simulink model "3_ZSM"  (R2016a)
settings: Solver=ode1  StartTime=0.0  StopTime=t_sim  FixedStep=0.001  RelTol=1e-3
values from neighbouring files (symbols this model uses):
  A = 1.5    [3_ZSM_Parameters.m]
  C = 1.3    [2_ESM_Parameters.m]    (also in 3_ZSM_Parameters.m)
  c_h_l = 0.5 * c_h    (= 71619.7243914)    [3_ZSM_Parameters.m]
  c_h_r = 0.5 * c_h    (= 71619.7243914)    [3_ZSM_Parameters.m]
  c_v_l = 0.5 * c_v    (= 39054.886799)    [3_ZSM_Parameters.m]
  c_v_r = 0.5 * c_v    (= 39054.886799)    [3_ZSM_Parameters.m]
  c_w = 0.4    [3_ZSM_Parameters.m]
  dynamicload_mode = i-1    [3_ZSM_Parameters.m]
  E = 0.85    [2_ESM_Parameters.m]    (also in 3_ZSM_Parameters.m)
  f_x_init = 0.5*A*c_w*rho*v_init^2    (= 24.980004)    [3_ZSM_Parameters.m]
  fz1 = fz(:,1)    [3_ZSM_Parameters.m]
  g = 9.81    [3_ZSM_Parameters.m]
  h_s = 0.5    [3_ZSM_Parameters.m]
  L = 2.71    [2_ESM_Parameters.m]    (also in 3_ZSM_Parameters.m)
  l_h = m_v * L / m    (= 1.35481930924)    [2_ESM_Parameters.m]    (also in 3_ZSM_Parameters.m)
  l_v = m_h * L / m    (= 1.35518069076)    [2_ESM_Parameters.m]    (also in 3_ZSM_Parameters.m)
  m = m_v + m_h    (= 1499.8)    [2_ESM_Parameters.m]    (also in 3_ZSM_Parameters.m)
  m_hl = m * l_v / L * SP_yl    (= 375)    [3_ZSM_Parameters.m]
  m_hr = m * l_v / L * SP_yr    (= 375)    [3_ZSM_Parameters.m]
  m_vl = m * l_h / L * SP_yl    (= 374.9)    [3_ZSM_Parameters.m]
  m_vr = m * l_h / L * SP_yr    (= 374.9)    [3_ZSM_Parameters.m]
  mu = 0.9    [2_ESM_Parameters.m]    (also in 3_ZSM_Parameters.m)
  rho = 1.2    [3_ZSM_Parameters.m]
  s_h = 1.57    [3_ZSM_Parameters.m]
  s_v = 1.54    [3_ZSM_Parameters.m]
  SP_yl = 0.5    [3_ZSM_Parameters.m]
  SP_yr = 1 - SP_yl    (= 0.5)    [3_ZSM_Parameters.m]
  v = setting(i,3)    [2_ESM_Parameters.m]
  v_init = 8.33    [3_ZSM_Parameters.m]
undefined symbols (not defined in the file or in its folder): Delta, fz
undefined symbols (not defined in the file): Lenkwinkel, Radlenkwinkel, T_z
libraries: simulink x2
(part 1 of 2)
settings Model: Creator=KFZ00  LastModifiedBy=Mario
settings DataIOCC: SaveFormat=Array  SaveOutput=off  TimeSaveName=t_out
settings DebuggingCC: AllowSymbolicDim=off
settings ModelReferenceCC: PropagateSignalLabelsOutOfModel=off
settings GRTTargetCC: GeneratePreprocessorConditionals=Use local settings

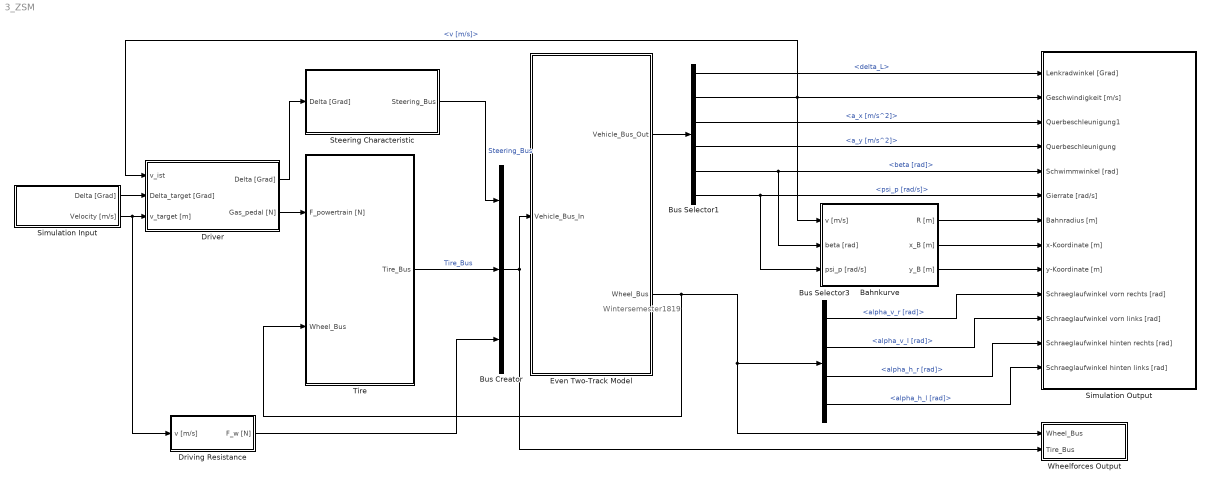
== system 3_ZSM ==
  note: Wintersemester1819
  Bahnkurve : Subsystem
  Bus Creator : BusCreator  Inputs=3
  Bus Selector1 : BusSelector  OutputSignals=delta_L,v [m/s],a_x [m/s^2],a_y [m/s^2],beta [rad],psi_p [rad/s]
  Bus Selector3 : BusSelector  OutputSignals=alpha_v_r [rad],alpha_v_l [rad],alpha_h_r [rad],alpha_h_l [rad]
  Driver : Subsystem
  Driving Resistance : Subsystem
  Even Two-Track Model : Subsystem  mask(Vehicle Model){m_body=m, I_zz_body=T_z, l_front=l_v, l_rear=l_h, tw_front=s_v, tw_rear=s_h, wb=L, h_cog=h_s, g=g}
      mask prompts: m_body "Vehicle Body Mass [kg]"; I_zz_body "Vehicle Body Inertia zz [kgm^2]"; l_front "Distance COG Front Axle [m]"; l_rear "Distance COG Rear Axle [m]"; tw_front "Track Width Front Axle [m]"; tw_rear "Track Width Rear Axle [m]"; wb "Wheelbase [m]"; h_cog "Height COG [m]"; g "Gravity [m/s^2]"
      mask help:
      | Even two-track model without wheel bodies and suspension system.
      |
      | Source for equations:
      | Von Vietinghoff, A.: Nichtlineare Regelung von Kraftfahrzeugen in
      | querdynamisch kritischen Fahrsituationen. Dissertation, Universität
      | Karlsruhe, S. 10 - 33, 2008.
  Simulation Input : Subsystem
  Simulation Output : Subsystem
  Steering Characteristic : Subsystem  mask(Steering Model){Input_values=Lenkwinkel, Steering_angles=Radlenkwinkel}
      mask prompts: Input_values "Steering Input Values [°]"; Steering_angles "Wheel Steer Angles [°]"
      mask help:
      | Steering model uses a look-up table to determine the current wheel
      | steer angle.
      | The steering angle of the rear wheel is set to zero!
      |
      | In order to configure the look-up table define the input values (steering
      | wheel angle in °) and the corresponding wheel steer angles (in °).
  Tire : Subsystem
  Wheelforces Output : Subsystem
  wires:
  Driver/1(Delta [Grad]) -> Steering Characteristic/1(Delta [Grad])
  Bus Creator/1 -> Even Two-Track Model/1(Vehicle_Bus_In), Wheelforces Output/2(Tire_Bus)
  Steering Characteristic/1(Steering_Bus) -> Bus Creator/1  "Steering_Bus"
  Tire/1(Tire_Bus) -> Bus Creator/2  "Tire_Bus"
  Even Two-Track Model/2(Wheel_Bus) -> Tire/2(Wheel_Bus), Bus Selector3/1, Wheelforces Output/1(Wheel_Bus)
  Even Two-Track Model/1(Vehicle_Bus_Out) -> Bus Selector1/1
  Bus Selector1/2 -> Bahnkurve/1(v [m/s]), Simulation Output/2(Geschwindigkeit [m/s]), Driver/1(v_ist)  "<v [m/s]>"
  Bus Selector1/4 -> Simulation Output/4(Querbeschleunigung)  "<a_y [m/s^2]>"
  Bus Selector1/5 -> Bahnkurve/2(beta [rad]), Simulation Output/5(Schwimmwinkel [rad])  "<beta [rad]>"
  Bus Selector1/6 -> Bahnkurve/3(psi_p [rad/s]), Simulation Output/6(Gierrate [rad/s])  "<psi_p [rad/s]>"
  Bus Selector3/1 -> Simulation Output/10(Schraeglaufwinkel vorn rechts [rad])  "<alpha_v_r [rad]>"
  Bus Selector3/2 -> Simulation Output/11(Schraeglaufwinkel vorn links [rad])  "<alpha_v_l [rad]>"
  Bus Selector3/3 -> Simulation Output/12(Schraeglaufwinkel hinten rechts [rad])  "<alpha_h_r [rad]>"
  Bus Selector3/4 -> Simulation Output/13(Schraeglaufwinkel hinten links [rad])  "<alpha_h_l [rad]>"
  Driving Resistance/1(F_w [N]) -> Bus Creator/3
  Bahnkurve/2(x_B [m]) -> Simulation Output/8(x-Koordinate [m])
  Bahnkurve/3(y_B [m]) -> Simulation Output/9(y-Koordinate [m])
  Bahnkurve/1(R [m]) -> Simulation Output/7(Bahnradius [m])
  Driver/2(Gas_pedal [N]) -> Tire/1(F_powertrain [N])
  Simulation Input/1(Delta [Grad]) -> Driver/2(Delta_target [Grad])
  Simulation Input/2(Velocity [m/s]) -> Driving Resistance/1(v [m/s]), Driver/3(v_target [m])
  Bus Selector1/1 -> Simulation Output/1(Lenkradwinkel [Grad])  "<delta_L>"
  Bus Selector1/3 -> Simulation Output/3(Querbeschleunigung1)  "<a_x [m/s^2]>"

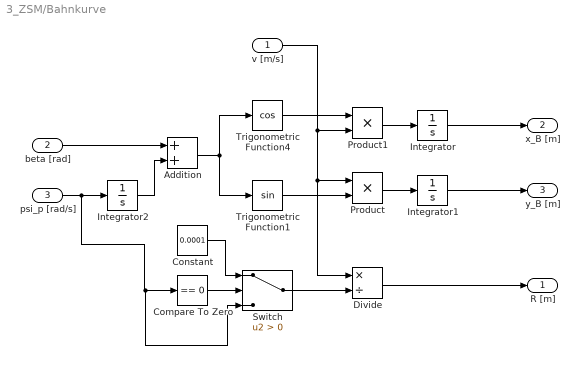
== system 3_ZSM/Bahnkurve ==
  v [m/s] : Inport
  beta [rad] : Inport  Port=2
  psi_p [rad/s] : Inport  Port=3
  Addition : Sum
  Compare To Zero : simulink/Logic and Bit Operations/Compare To Zero  relop===  OutDataTypeStr=boolean
  Constant : Constant  Value=0.0001
  Divide : Product  Inputs=*/
  Integrator : Integrator
  Integrator1 : Integrator
  Integrator2 : Integrator
  Product : Product
  Product1 : Product
  Switch : Switch  Criteria=u2 > Threshold
  Trigonometric Function1 : Trigonometry
  Trigonometric Function4 : Trigonometry  Operator=cos
  R [m] : Outport
  x_B [m] : Outport  Port=2
  y_B [m] : Outport  Port=3
  wires:
  Trigonometric Function4/1 -> Product1/1
  Trigonometric Function1/1 -> Product/2
  Product/1 -> Integrator1/1
  Addition/1 -> Trigonometric Function1/1, Trigonometric Function4/1
  psi_p [rad/s]/1 -> Integrator2/1, Switch/3, Compare To Zero/1
  Integrator2/1 -> Addition/2
  Product1/1 -> Integrator/1
  v [m/s]/1 -> Divide/1, Product/1, Product1/2
  Integrator/1 -> x_B [m]/1
  Integrator1/1 -> y_B [m]/1
  beta [rad]/1 -> Addition/1
  Switch/1 -> Divide/2
  Compare To Zero/1 -> Switch/2
  Divide/1 -> R [m]/1
  Constant/1 -> Switch/1

== system 3_ZSM/Driver ==
  v_ist : Inport
  Delta_target [Grad] : Inport  Port=2
  v_target [m] : Inport  Port=3
  Constant : Constant  Value=f_x_init
  P_Fx : simulink/Continuous/PID Controller (2DOF)  Controller=PI  TimeDomain=Continuous-time  SampleTime=-1  IntegratorMethod=Forward Euler  FilterMethod=Forward Euler  Form=Parallel  UseFilter=on  ControllerParametersSource=internal  P=100000  I=0  D=0  N=100  b=1  c=1  InitialConditionSource=external  InitialConditionForIntegrator=0  InitialConditionForFilter=0  ExternalReset=none  LimitOutput=off  UpperSaturationLimit=9000  LowerSaturationLimit=0  LinearizeAsGain=on  AntiWindupMode=none  Kb=1  TrackingMode=off  Kt=1  PParamMin=[]  PParamMax=[]  IParamMin=[]  IParamMax=[]  DParamMin=[]  DParamMax=[]  NParamMin=[]  NParamMax=[]  bParamMin=[]  bParamMax=[]  cParamMin=[]  cParamMax=[]  KbParamMin=[]  KbParamMax=[]  KtParamMin=[]  KtParamMax=[]  POutMin=[]  POutMax=[]  IOutMin=[]  IOutMax=[]  DOutMin=[]  DOutMax=[]  NOutMin=[]  NOutMax=[]  bOutMin=[]  bOutMax=[]  cOutMin=[]  cOutMax=[]  KbOutMin=[]  KbOutMax=[]  KtOutMin=[]  KtOutMax=[]  IntegratorOutMin=[]  IntegratorOutMax=[]  FilterOutMin=[]  FilterOutMax=[]  SumOutMin=[]  SumOutMax=[]  Sum1OutMin=[]  Sum1OutMax=[]  Sum2OutMin=[]  Sum2OutMax=[]  Sum3OutMin=[]  Sum3OutMax=[]  SumI1OutMin=[]  SumI1OutMax=[]  SumI2OutMin=[]  SumI2OutMax=[]  SumI3OutMin=[]  SumI3OutMax=[]  SumDOutMin=[]  SumDOutMax=[]  SaturationOutMin=[]  SaturationOutMax=[]  IntegratorContinuousStateAttributes=''  IntegratorStateMustResolveToSignalObject=off  IntegratorRTWStateStorageClass=Auto  FilterContinuousStateAttributes=''  FilterStateMustResolveToSignalObject=off  FilterRTWStateStorageClass=Auto  DifferentiatorICPrevScaledInput=0  DifferentiatorOutMin=[]  DifferentiatorOutMax=[]
  Scope : Scope  NumInputPorts=2
  Delta [Grad] : Outport
  Gas_pedal [N] : Outport  Port=2
  wires:
  v_target [m]/1 -> Scope/1, P_Fx/1
  Constant/1 -> P_Fx/3
  P_Fx/1 -> Gas_pedal [N]/1
  v_ist/1 -> Scope/2, P_Fx/2
  Delta_target [Grad]/1 -> Delta [Grad]/1

== system 3_ZSM/Driving Resistance ==
  v [m/s] : Inport
  Constant : Constant  Value=c_w
  Constant1 : Constant  Value=A
  Constant2 : Constant  Value=rho
  Constant3 : Constant  Value=0.5
  Math Function : Math  Operator=square  SaturateOnIntegerOverflow=on
  Product : Product  Inputs=5
  F_w [N] : Outport
  wires:
  Constant3/1 -> Product/5
  Product/1 -> F_w [N]/1  "Driving_resistance [N]"
  Constant2/1 -> Product/4
  Constant/1 -> Product/1
  v [m/s]/1 -> Math Function/1
  Math Function/1 -> Product/3
  Constant1/1 -> Product/2

== system 3_ZSM/Even Two-Track Model ==
  Vehicle_Bus_In : Inport
  Bus Creator1 : BusCreator  Inputs=8
  Bus Creator2 : BusCreator  Inputs=6
  Bus Selector : BusSelector  OutputSignals=Steering_Bus.delta_L
  Calculate Wheel Load : Subsystem
  Calculate forces on vehicle body : Subsystem
  Calculate side slip angle : Subsystem
  Calculate sum of forces (x and y) : Subsystem
  Calculate velocity : Subsystem
  Calculate yaw rate : Subsystem
  Determine vehicle body movement in vehicle COS : Subsystem
  Determine wheel movement : Subsystem
  Scope : Scope
  Vehicle_Bus_Out : Outport
  Wheel_Bus : Outport  Port=2
  wires:
  Calculate velocity/1(v [m/s]) -> Determine vehicle body movement in vehicle COS/1(v [m/s]), Calculate side slip angle/1(v [m/s]), Bus Creator2/3, Determine wheel movement/1(vehicle_velocity [m/s])  "v [m/s]"
  Determine vehicle body movement in vehicle COS/2(a_y [m/s^2]) -> Calculate Wheel Load/2(a_y [m/s²]), Bus Creator2/2  "a_y [m/s^2]"
  Calculate side slip angle/2(beta_p [rad/s]) -> Scope/1, Determine vehicle body movement in vehicle COS/4(beta_p [rad/s])
  Calculate velocity/2(v_p [m/s^2]) -> Determine vehicle body movement in vehicle COS/2(v_p [m/s^2])
  Calculate sum of forces (x and y)/2(Sum_F_y [N]) -> Calculate velocity/2(Sum_F_y [N]), Calculate side slip angle/3(Sum_F_y [N])
  Calculate sum of forces (x and y)/1(Sum_F_x [N]) -> Calculate side slip angle/2(Sum_F_x [N]), Calculate velocity/1(Sum_F_x [N])
  Calculate side slip angle/1(Side_slip_angle [rad]) -> Determine vehicle body movement in vehicle COS/3(beta [rad]), Calculate side slip angle/4(beta [rad]), Calculate velocity/3(beta [rad]), Bus Creator2/4, Determine wheel movement/2(beta [rad])  "beta [rad]"
  Calculate forces on vehicle body/1(Forces_vehicle_COS [N]) -> Calculate sum of forces (x and y)/1(Forces_vehicle_body [N]), Calculate yaw rate/1(Forces_vehicle_body [N])
  Calculate yaw rate/1(psi_p [rad/s]) -> Determine vehicle body movement in vehicle COS/5(psi_p [rad/s]), Calculate side slip angle/5(psi_p [rad]), Bus Creator2/5, Determine wheel movement/3(psi_p [rad/s])  "psi_p [rad/s]"
  Vehicle_Bus_In/1 -> Calculate forces on vehicle body/1(Vehicle Bus), Determine wheel movement/4(Vehicle Bus In), Bus Selector/1
  Bus Creator1/1 -> Wheel_Bus/1
  Bus Creator2/1 -> Vehicle_Bus_Out/1
  Determine vehicle body movement in vehicle COS/1(a_x [m/s^2]) -> Bus Creator2/1, Calculate Wheel Load/1(a_x [m/s²])  "a_x [m/s^2]"
  Calculate Wheel Load/1(F_z_v_l [N]) -> Bus Creator1/1  "F_z_v_l [N]"
  Calculate Wheel Load/2(F_z_v_r [N]) -> Bus Creator1/2  "F_z_v_r [N]"
  Calculate Wheel Load/3(F_z_h_l [N]) -> Bus Creator1/3  "F_z_h_l [N]"
  Calculate Wheel Load/4(F_z_h_r [N]) -> Bus Creator1/4  "F_z_h_r [N]"
  Determine wheel movement/4(alpha_rear_left [rad]) -> Bus Creator1/8  "alpha_h_l [rad]"
  Determine wheel movement/3(alpha_rear_right [rad]) -> Bus Creator1/7  "alpha_h_r [rad]"
  Determine wheel movement/2(alpha_front_left [rad]) -> Bus Creator1/6  "alpha_v_l [rad]"
  Determine wheel movement/1(alpha_front_right [rad]) -> Bus Creator1/5  "alpha_v_r [rad]"
  Bus Selector/1 -> Bus Creator2/6  "<delta_L>"

== system 3_ZSM/Simulation Input ==
  1-D Lookup Table : Lookup_n-D  NumberOfTableDimensions=1  BreakpointsForDimension1=Delta.time  Table=Delta.signals.values  InternalRulePriority=Speed  RndMeth=Simplest  InputSameDT=on
  1-D Lookup Table1 : Lookup_n-D  NumberOfTableDimensions=1  BreakpointsForDimension1=v.time  Table=v.signals.values  InternalRulePriority=Speed  RndMeth=Simplest  InputSameDT=on
  Clock : Clock
  Gain : Gain  Gain=1/3.6
  Delta [Grad] : Outport
  Velocity [m/s] : Outport  Port=2
  wires:
  Clock/1 -> 1-D Lookup Table/1, 1-D Lookup Table1/1
  1-D Lookup Table/1 -> Delta [Grad]/1
  1-D Lookup Table1/1 -> Gain/1
  Gain/1 -> Velocity [m/s]/1

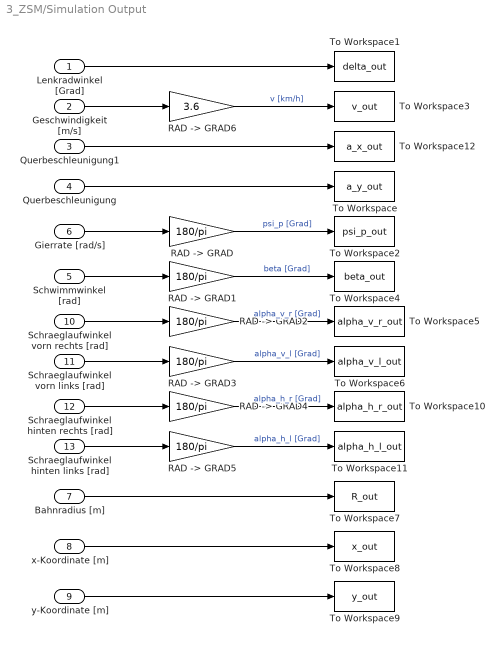
== system 3_ZSM/Simulation Output ==
  Lenkradwinkel [Grad] : Inport
  Geschwindigkeit [m/s] : Inport  Port=2
  Querbeschleunigung1 : Inport  Port=3
  Querbeschleunigung : Inport  Port=4
  Schwimmwinkel [rad] : Inport  Port=5
  Gierrate [rad/s] : Inport  Port=6
  Bahnradius [m] : Inport  Port=7
  x-Koordinate [m] : Inport  Port=8
  y-Koordinate [m] : Inport  Port=9
  Schraeglaufwinkel vorn rechts [rad] : Inport  Port=10
  Schraeglaufwinkel vorn links [rad] : Inport  Port=11
  Schraeglaufwinkel hinten rechts [rad] : Inport  Port=12
  Schraeglaufwinkel hinten links [rad] : Inport  Port=13
  RAD -> GRAD{,1..5} (6 alike) : Gain  Gain=180/pi
  "RAD -> GRAD6" : Gain  Gain=3.6
  To Workspace : ToWorkspace  VariableName=a_y_out  SampleTime=-1
      settings: Save2DSignal=2-D array (concatenate along first dimension)
  To Workspace1 : ToWorkspace  VariableName=delta_out  SampleTime=-1
      settings: Save2DSignal=2-D array (concatenate along first dimension)
  To Workspace10 : ToWorkspace  VariableName=alpha_h_r_out  SampleTime=-1
      settings: Save2DSignal=2-D array (concatenate along first dimension)
  To Workspace11 : ToWorkspace  VariableName=alpha_h_l_out  SampleTime=-1
      settings: Save2DSignal=2-D array (concatenate along first dimension)
  To Workspace12 : ToWorkspace  VariableName=a_x_out  SampleTime=-1
      settings: Save2DSignal=2-D array (concatenate along first dimension)
  To Workspace2 : ToWorkspace  VariableName=psi_p_out  SampleTime=-1
      settings: Save2DSignal=2-D array (concatenate along first dimension)
  To Workspace3 : ToWorkspace  VariableName=v_out  SampleTime=-1
      settings: Save2DSignal=2-D array (concatenate along first dimension)
  To Workspace4 : ToWorkspace  VariableName=beta_out  SampleTime=-1
      settings: Save2DSignal=2-D array (concatenate along first dimension)
  To Workspace5 : ToWorkspace  VariableName=alpha_v_r_out  SampleTime=-1
      settings: Save2DSignal=2-D array (concatenate along first dimension)
  To Workspace6 : ToWorkspace  VariableName=alpha_v_l_out  SampleTime=-1
      settings: Save2DSignal=2-D array (concatenate along first dimension)
  To Workspace7 : ToWorkspace  VariableName=R_out  SampleTime=-1
      settings: Save2DSignal=2-D array (concatenate along first dimension)
  To Workspace8 : ToWorkspace  VariableName=x_out  SampleTime=-1
      settings: Save2DSignal=2-D array (concatenate along first dimension)
  To Workspace9 : ToWorkspace  VariableName=y_out  SampleTime=-1
      settings: Save2DSignal=2-D array (concatenate along first dimension)
  wires:
  Gierrate [rad/s]/1 -> "RAD -> GRAD"/1
  "RAD -> GRAD"/1 -> To Workspace2/1  "psi_p [Grad]"
  Lenkradwinkel [Grad]/1 -> To Workspace1/1
  Geschwindigkeit [m/s]/1 -> "RAD -> GRAD6"/1
  Schwimmwinkel [rad]/1 -> "RAD -> GRAD1"/1
  "RAD -> GRAD1"/1 -> To Workspace4/1  "beta [Grad]"
  Schraeglaufwinkel vorn rechts [rad]/1 -> "RAD -> GRAD2"/1
  "RAD -> GRAD2"/1 -> To Workspace5/1  "alpha_v_r [Grad]"
  Schraeglaufwinkel vorn links [rad]/1 -> "RAD -> GRAD3"/1
  "RAD -> GRAD3"/1 -> To Workspace6/1  "alpha_v_l [Grad]"
  Bahnradius [m]/1 -> To Workspace7/1
  x-Koordinate [m]/1 -> To Workspace8/1
  y-Koordinate [m]/1 -> To Workspace9/1
  Schraeglaufwinkel hinten rechts [rad]/1 -> "RAD -> GRAD4"/1
  "RAD -> GRAD4"/1 -> To Workspace10/1  "alpha_h_r [Grad]"
  Schraeglaufwinkel hinten links [rad]/1 -> "RAD -> GRAD5"/1
  "RAD -> GRAD5"/1 -> To Workspace11/1  "alpha_h_l [Grad]"
  "RAD -> GRAD6"/1 -> To Workspace3/1  "v [km/h]"
  Querbeschleunigung/1 -> To Workspace/1
  Querbeschleunigung1/1 -> To Workspace12/1

== system 3_ZSM/Steering Characteristic ==
  Delta [Grad] : Inport  OutDataTypeStr=double
  1-D Lookup Table : Lookup_n-D  NumberOfTableDimensions=1  BreakpointsForDimension1=Input_values  Table=Steering_angles  InternalRulePriority=Speed  RndMeth=Simplest  InputSameDT=on
  Bus Creator : BusCreator  Inputs=5
  "Grad -> RAD1" : Gain  Gain=pi/180
  "Grad -> RAD2" : Gain  Gain=pi/180
  Rear wheel steering left : Constant  Value=0
  Rear wheel steering right : Constant  Value=0
  Steering_Bus : Outport  OutDataTypeStr=double
  wires:
  Bus Creator/1 -> Steering_Bus/1
  1-D Lookup Table/1 -> "Grad -> RAD1"/1, "Grad -> RAD2"/1
  "Grad -> RAD1"/1 -> Bus Creator/1  "Delta_v_l"
  "Grad -> RAD2"/1 -> Bus Creator/2  "Delta_v_r"
  Rear wheel steering left/1 -> Bus Creator/3  "Delta_h_l"
  Rear wheel steering right/1 -> Bus Creator/4  "Delta_h_r"
  Delta [Grad]/1 -> Bus Creator/5, 1-D Lookup Table/1  "delta_L"

== system 3_ZSM/Tire ==
  F_powertrain [N] : Inport
  Wheel_Bus : Inport  Port=2
  Bus Creator : BusCreator  Inputs=4
  Constant : Constant  Value=mu
  Constant1 : Constant  Value=0
  Gain : Gain  Gain=1/2
  Tire front left : Subsystem
  Tire front right : Subsystem
  Tire rear left : Subsystem
  Tire rear right : Subsystem
  Tire_Bus : Outport
  wires:
  F_powertrain [N]/1 -> Gain/1
  Bus Creator/1 -> Tire_Bus/1
  Wheel_Bus/1 -> Tire rear right/2(Wheel_Bus), Tire rear left/2(Wheel_Bus), Tire front right/2(Wheel_Bus), Tire front left/2(Wheel_Bus)
  Tire rear right/1(Tire_front_left) -> Bus Creator/4  "Tire_rear_right"
  Tire rear left/1(Tire_rear_left) -> Bus Creator/3  "Tire_rear_left"
  Tire front right/1(Tire_front_right) -> Bus Creator/2  "Tire_front_right"
  Tire front left/1(Tire_front_left) -> Bus Creator/1  "Tire_front_left"
  Constant/1 -> Tire front right/3(nu_v_r [-]), Tire rear left/3(nu_h_l [-]), Tire rear right/3(nu_h_r [-]), Tire front left/3(nu_v_l [-])
  Constant1/1 -> Tire rear left/1(F_powertrain [N]), Tire rear right/1(F_powertrain [N])
  Gain/1 -> Tire front right/1(F_powertrain [N]), Tire front left/1(F_powertrain [N])

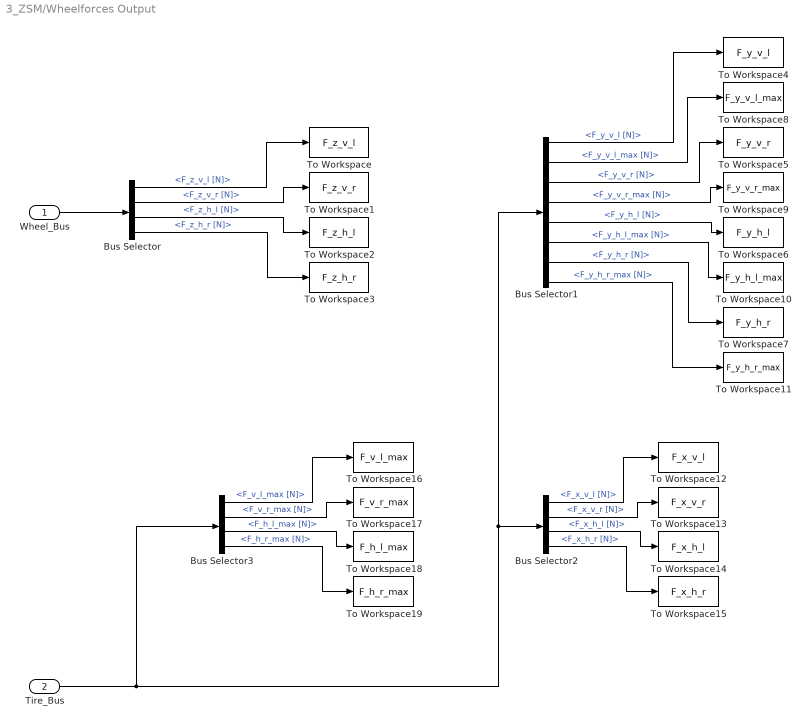
== system 3_ZSM/Wheelforces Output ==
  Wheel_Bus : Inport
  Tire_Bus : Inport  Port=2
  Bus Selector : BusSelector  OutputSignals=F_z_v_l [N],F_z_v_r [N],F_z_h_l [N],F_z_h_r [N]
  Bus Selector1 : BusSelector  OutputSignals=Tire_Bus.Tire_front_left.F_y_v_l [N],Tire_Bus.Tire_front_left.F_y_v_l_max [N],Tire_Bus.Tire_front_right.F_y_v_r [N],Tire_Bus.Tire_front_right.F_y_v_r_max [N],Tire_Bus.Tire_rear_left.F_y_h_l [N],Tire_Bus.Tire_rear_left.F_y_h_l_max [N],Tire_Bus.Tire_rear_right.F_y_h_r [N],Tire_Bus.Tire_rear_right.F_y_h_r_max [N]
  Bus Selector2 : BusSelector  OutputSignals=Tire_Bus.Tire_front_left.F_x_v_l [N],Tire_Bus.Tire_front_right.F_x_v_r [N],Tire_Bus.Tire_rear_left.F_x_h_l [N],Tire_Bus.Tire_rear_right.F_x_h_r [N]
  Bus Selector3 : BusSelector  OutputSignals=Tire_Bus.Tire_front_left.F_v_l_max [N],Tire_Bus.Tire_front_right.F_v_r_max [N],Tire_Bus.Tire_rear_left.F_h_l_max [N],Tire_Bus.Tire_rear_right.F_h_r_max [N]
  To Workspace : ToWorkspace  VariableName=F_z_v_l  SampleTime=-1
      settings: Save2DSignal=2-D array (concatenate along first dimension)
  To Workspace1 : ToWorkspace  VariableName=F_z_v_r  SampleTime=-1
      settings: Save2DSignal=2-D array (concatenate along first dimension)
  To Workspace10 : ToWorkspace  VariableName=F_y_h_l_max  SampleTime=-1
      settings: Save2DSignal=2-D array (concatenate along first dimension)
  To Workspace11 : ToWorkspace  VariableName=F_y_h_r_max  SampleTime=-1
      settings: Save2DSignal=2-D array (concatenate along first dimension)
  To Workspace12 : ToWorkspace  VariableName=F_x_v_l  SampleTime=-1
      settings: Save2DSignal=2-D array (concatenate along first dimension)
  To Workspace13 : ToWorkspace  VariableName=F_x_v_r  SampleTime=-1
      settings: Save2DSignal=2-D array (concatenate along first dimension)
  To Workspace14 : ToWorkspace  VariableName=F_x_h_l  SampleTime=-1
      settings: Save2DSignal=2-D array (concatenate along first dimension)
  To Workspace15 : ToWorkspace  VariableName=F_x_h_r  SampleTime=-1
      settings: Save2DSignal=2-D array (concatenate along first dimension)
  To Workspace16 : ToWorkspace  VariableName=F_v_l_max  SampleTime=-1
      settings: Save2DSignal=2-D array (concatenate along first dimension)
  To Workspace17 : ToWorkspace  VariableName=F_v_r_max  SampleTime=-1
      settings: Save2DSignal=2-D array (concatenate along first dimension)
  To Workspace18 : ToWorkspace  VariableName=F_h_l_max  SampleTime=-1
      settings: Save2DSignal=2-D array (concatenate along first dimension)
  To Workspace19 : ToWorkspace  VariableName=F_h_r_max  SampleTime=-1
      settings: Save2DSignal=2-D array (concatenate along first dimension)
  To Workspace2 : ToWorkspace  VariableName=F_z_h_l  SampleTime=-1
      settings: Save2DSignal=2-D array (concatenate along first dimension)
  To Workspace3 : ToWorkspace  VariableName=F_z_h_r  SampleTime=-1
      settings: Save2DSignal=2-D array (concatenate along first dimension)
  To Workspace4 : ToWorkspace  VariableName=F_y_v_l  SampleTime=-1
      settings: Save2DSignal=2-D array (concatenate along first dimension)
  To Workspace5 : ToWorkspace  VariableName=F_y_v_r  SampleTime=-1
      settings: Save2DSignal=2-D array (concatenate along first dimension)
  To Workspace6 : ToWorkspace  VariableName=F_y_h_l  SampleTime=-1
      settings: Save2DSignal=2-D array (concatenate along first dimension)
  To Workspace7 : ToWorkspace  VariableName=F_y_h_r  SampleTime=-1
      settings: Save2DSignal=2-D array (concatenate along first dimension)
  To Workspace8 : ToWorkspace  VariableName=F_y_v_l_max  SampleTime=-1
      settings: Save2DSignal=2-D array (concatenate along first dimension)
  To Workspace9 : ToWorkspace  VariableName=F_y_v_r_max  SampleTime=-1
      settings: Save2DSignal=2-D array (concatenate along first dimension)
  wires:
  Wheel_Bus/1 -> Bus Selector/1
  Bus Selector/1 -> To Workspace/1  "<F_z_v_l [N]>"
  Bus Selector/2 -> To Workspace1/1  "<F_z_v_r [N]>"
  Bus Selector/3 -> To Workspace2/1  "<F_z_h_l [N]>"
  Bus Selector/4 -> To Workspace3/1  "<F_z_h_r [N]>"
  Bus Selector1/1 -> To Workspace4/1  "<F_y_v_l [N]>"
  Bus Selector1/7 -> To Workspace7/1  "<F_y_h_r [N]>"
  Bus Selector1/3 -> To Workspace5/1  "<F_y_v_r [N]>"
  Bus Selector1/4 -> To Workspace9/1  "<F_y_v_r_max [N]>"
  Bus Selector1/8 -> To Workspace11/1  "<F_y_h_r_max [N]>"
  Bus Selector1/2 -> To Workspace8/1  "<F_y_v_l_max [N]>"
  Bus Selector1/5 -> To Workspace6/1  "<F_y_h_l [N]>"
  Bus Selector1/6 -> To Workspace10/1  "<F_y_h_l_max [N]>"
  Tire_Bus/1 -> Bus Selector3/1, Bus Selector2/1, Bus Selector1/1
  Bus Selector2/1 -> To Workspace12/1  "<F_x_v_l [N]>"
  Bus Selector2/2 -> To Workspace13/1  "<F_x_v_r [N]>"
  Bus Selector2/3 -> To Workspace14/1  "<F_x_h_l [N]>"
  Bus Selector2/4 -> To Workspace15/1  "<F_x_h_r [N]>"
  Bus Selector3/1 -> To Workspace16/1  "<F_v_l_max [N]>"
  Bus Selector3/2 -> To Workspace17/1  "<F_v_r_max [N]>"
  Bus Selector3/3 -> To Workspace18/1  "<F_h_l_max [N]>"
  Bus Selector3/4 -> To Workspace19/1  "<F_h_r_max [N]>"

== system 3_ZSM/Even Two-Track Model/Calculate Wheel Load ==
  a_x [m/s²] : Inport
  a_y [m/s²] : Inport  Port=2
  Dynamic Wheel Load : Subsystem
  Load_Mode : Constant  Value=dynamicload_mode
  Scope : Scope
  Static Wheel Load : Subsystem
  Switch{,1..3} (4 alike) : Switch  Criteria=u2 > Threshold
  F_z_v_l [N] : Outport
  F_z_v_r [N] : Outport  Port=2
  F_z_h_l [N] : Outport  Port=3
  F_z_h_r [N] : Outport  Port=4
  wires:
  a_x [m/s²]/1 -> Dynamic Wheel Load/1(a_x [m/s²])
  a_y [m/s²]/1 -> Dynamic Wheel Load/2(a_y [m/s²])
  Switch/1 -> Scope/1, F_z_v_l [N]/1
  Switch1/1 -> F_z_v_r [N]/1
  Switch2/1 -> F_z_h_l [N]/1
  Switch3/1 -> F_z_h_r [N]/1
  Dynamic Wheel Load/1(F_z_v_l [N]) -> Switch/1
  Dynamic Wheel Load/2(F_z_v_r [N]) -> Switch1/1
  Dynamic Wheel Load/3(F_z_h_l [N]) -> Switch2/1
  Dynamic Wheel Load/4(F_z_h_r [N]) -> Switch3/1
  Static Wheel Load/1(F_z_v_l [N]) -> Switch/3
  Static Wheel Load/2(F_z_v_r [N]) -> Switch1/3
  Static Wheel Load/3(F_z_h_l [N]) -> Switch2/3
  Static Wheel Load/4(F_z_h_r [N]) -> Switch3/3
  Load_Mode/1 -> Switch1/2, Switch3/2, Switch2/2, Switch/2

== system 3_ZSM/Even Two-Track Model/Calculate forces on vehicle body ==
  Vehicle Bus : Inport
  Bus Creator1 : BusCreator  Inputs=9
  Bus Selector : BusSelector  OutputSignals=Driving_resistance [N],Tire_Bus.Tire_front_right,Steering_Bus.Delta_v_r,Tire_Bus.Tire_front_left,Steering_Bus.Delta_v_l,Tire_Bus.Tire_rear_right,Steering_Bus.Delta_h_r,Tire_Bus.Tire_rear_left,Steering_Bus.Delta_h_l
  Bus Selector1 : BusSelector  OutputSignals=F_x_v_r [N],F_y_v_r [N]
  Bus Selector2 : BusSelector  OutputSignals=F_x_v_l [N],F_y_v_l [N]
  Bus Selector3 : BusSelector  OutputSignals=F_x_h_r [N],F_y_h_r [N]
  Bus Selector4 : BusSelector  OutputSignals=F_x_h_l [N],F_y_h_l [N]
  Transform Wheel-COS to Vehicle-COS (front left) : Subsystem
  Transform Wheel-COS to Vehicle-COS (front right) : Subsystem
  Transform Wheel-COS to Vehicle-COS (rear left) : Subsystem
  Transform Wheel-COS to Vehicle-COS (rear right) : Subsystem
  Forces_vehicle_COS [N] : Outport
  wires:
  Vehicle Bus/1 -> Bus Selector/1
  Bus Creator1/1 -> Forces_vehicle_COS [N]/1
  Bus Selector1/1 -> Transform Wheel-COS to Vehicle-COS (front right)/1(F_x_wheel_COS [N])  "<F_x_v_r [N]>"
  Transform Wheel-COS to Vehicle-COS (front left)/1(F_x_vehicle_COS [N]) -> Bus Creator1/4  "F_x_front_left [N]"
  Bus Selector4/2 -> Transform Wheel-COS to Vehicle-COS (rear left)/2(F_y_wheel_COS [N])  "<F_y_h_l [N]>"
  Transform Wheel-COS to Vehicle-COS (rear left)/2(F_y_vehicle_COS [N]) -> Bus Creator1/9  "F_y_rear_left [N]"
  Bus Selector/9 -> Transform Wheel-COS to Vehicle-COS (rear left)/3(Wheel_steering_angle [rad])  "<Delta_h_l>"
  Bus Selector/2 -> Bus Selector1/1  "<Tire_front_right>"
  Bus Selector4/1 -> Transform Wheel-COS to Vehicle-COS (rear left)/1(F_x_wheel_COS [N])  "<F_x_h_l [N]>"
  Bus Selector3/1 -> Transform Wheel-COS to Vehicle-COS (rear right)/1(F_x_wheel_COS [N])  "<F_x_h_r [N]>"
  Transform Wheel-COS to Vehicle-COS (rear right)/2(F_y_vehicle_COS [N]) -> Bus Creator1/7  "F_y_rear_right [N]"
  Bus Selector/7 -> Transform Wheel-COS to Vehicle-COS (rear right)/3(Wheel_steering_angle [rad])  "<Delta_h_r>"
  Bus Selector/4 -> Bus Selector2/1  "<Tire_front_left>"
  Transform Wheel-COS to Vehicle-COS (front left)/2(F_y_vehicle_COS [N]) -> Bus Creator1/5  "F_y_front_left [N]"
  Bus Selector3/2 -> Transform Wheel-COS to Vehicle-COS (rear right)/2(F_y_wheel_COS [N])  "<F_y_h_r [N]>"
  Bus Selector/5 -> Transform Wheel-COS to Vehicle-COS (front left)/3(Wheel_steering_angle [rad])  "<Delta_v_l>"
  Bus Selector/3 -> Transform Wheel-COS to Vehicle-COS (front right)/3(Wheel_steering_angle [rad])  "<Delta_v_r>"
  Transform Wheel-COS to Vehicle-COS (rear left)/1(F_x_vehicle_COS [N]) -> Bus Creator1/8  "F_x_rear_left [N]"
  Transform Wheel-COS to Vehicle-COS (front right)/1(F_x_vehicle_COS [N]) -> Bus Creator1/2  "F_x_front_right [N]"
  Transform Wheel-COS to Vehicle-COS (rear right)/1(F_x_vehicle_COS [N]) -> Bus Creator1/6  "F_x_rear_right [N]"
  Bus Selector/1 -> Bus Creator1/1  "<Driving_resistance [N]>"
  Bus Selector2/2 -> Transform Wheel-COS to Vehicle-COS (front left)/2(F_y_wheel_COS [N])  "<F_y_v_l [N]>"
  Bus Selector/8 -> Bus Selector4/1  "<Tire_rear_left>"
  Transform Wheel-COS to Vehicle-COS (front right)/2(F_y_vehicle_COS [N]) -> Bus Creator1/3  "F_y_front_right [N]"
  Bus Selector/6 -> Bus Selector3/1  "<Tire_rear_right>"
  Bus Selector1/2 -> Transform Wheel-COS to Vehicle-COS (front right)/2(F_y_wheel_COS [N])  "<F_y_v_r [N]>"
  Bus Selector2/1 -> Transform Wheel-COS to Vehicle-COS (front left)/1(F_x_wheel_COS [N])  "<F_x_v_l [N]>"

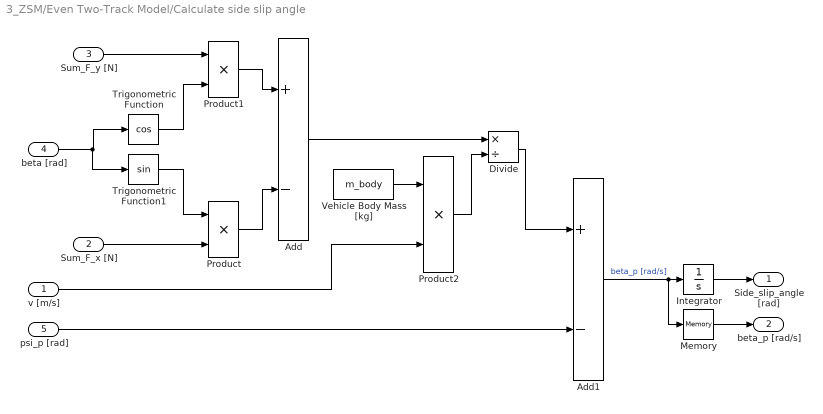
== system 3_ZSM/Even Two-Track Model/Calculate side slip angle ==
  v [m/s] : Inport
  Sum_F_x [N] : Inport  Port=2
  Sum_F_y [N] : Inport  Port=3
  beta [rad] : Inport  Port=4
  psi_p [rad] : Inport  Port=5
  Add : Sum  Inputs=+-
  Add1 : Sum  Inputs=+-
  Divide : Product  Inputs=*/
  Integrator : Integrator
  Memory : Memory
  Product : Product
  Product1 : Product
  Product2 : Product
  Trigonometric Function : Trigonometry  Operator=cos
  Trigonometric Function1 : Trigonometry
  Vehicle Body Mass [kg] : Constant  Value=m_body
  Side_slip_angle [rad] : Outport
  beta_p [rad/s] : Outport  Port=2
  wires:
  Memory/1 -> beta_p [rad/s]/1
  v [m/s]/1 -> Product2/2
  Product2/1 -> Divide/2
  Vehicle Body Mass [kg]/1 -> Product2/1
  Sum_F_y [N]/1 -> Product1/1
  Sum_F_x [N]/1 -> Product/2
  Add1/1 -> Integrator/1, Memory/1  "beta_p [rad/s]"
  psi_p [rad]/1 -> Add1/2
  Divide/1 -> Add1/1
  Integrator/1 -> Side_slip_angle [rad]/1
  Product/1 -> Add/2
  Trigonometric Function1/1 -> Product/1
  Product1/1 -> Add/1
  Trigonometric Function/1 -> Product1/2
  beta [rad]/1 -> Trigonometric Function/1, Trigonometric Function1/1
  Add/1 -> Divide/1

== system 3_ZSM/Even Two-Track Model/Calculate sum of forces (x and y) ==
  Forces_vehicle_body [N] : Inport
  Add : Sum  Inputs=-++++
  Add1 : Sum  Inputs=++++
  Bus Selector : BusSelector  OutputSignals=Driving_resistance [N],F_x_front_right [N],F_x_front_left [N],F_x_rear_right [N],F_x_rear_left [N]
  Bus Selector1 : BusSelector  OutputSignals=F_y_front_right [N],F_y_front_left [N],F_y_rear_right [N],F_y_rear_left [N]
  Memory : Memory
  Memory1 : Memory
  Sum_F_x [N] : Outport
  Sum_F_y [N] : Outport  Port=2
  wires:
  Add/1 -> Memory/1
  Add1/1 -> Memory1/1
  Bus Selector1/4 -> Add1/4  "<F_y_rear_left [N]>"
  Bus Selector1/3 -> Add1/3  "<F_y_rear_right [N]>"
  Bus Selector1/2 -> Add1/2  "<F_y_front_left [N]>"
  Bus Selector1/1 -> Add1/1  "<F_y_front_right [N]>"
  Bus Selector/5 -> Add/5  "<F_x_rear_left [N]>"
  Bus Selector/4 -> Add/4  "<F_x_rear_right [N]>"
  Bus Selector/3 -> Add/3  "<F_x_front_left [N]>"
  Bus Selector/2 -> Add/2  "<F_x_front_right [N]>"
  Bus Selector/1 -> Add/1  "<Driving_resistance [N]>"
  Forces_vehicle_body [N]/1 -> Bus Selector/1, Bus Selector1/1
  Memory/1 -> Sum_F_x [N]/1
  Memory1/1 -> Sum_F_y [N]/1

== system 3_ZSM/Even Two-Track Model/Calculate velocity ==
  Sum_F_x [N] : Inport
  Sum_F_y [N] : Inport  Port=2
  beta [rad] : Inport  Port=3
  Add : Sum
  Divide : Product  Inputs=*/
  Integrator : Integrator  InitialCondition=v_init
  Product : Product
  Product1 : Product
  Trigonometric Function : Trigonometry  Operator=cos
  Trigonometric Function1 : Trigonometry
  Vehicle Body Mass [kg] : Constant  Value=m_body
  v [m/s] : Outport
  v_p [m/s^2] : Outport  Port=2
  wires:
  Integrator/1 -> v [m/s]/1
  Divide/1 -> v_p [m/s^2]/1, Integrator/1  "v_p [m/s^2]"
  Product/1 -> Add/2
  Trigonometric Function1/1 -> Product/1
  Product1/1 -> Add/1
  Trigonometric Function/1 -> Product1/2
  beta [rad]/1 -> Trigonometric Function/1, Trigonometric Function1/1
  Sum_F_y [N]/1 -> Product/2
  Vehicle Body Mass [kg]/1 -> Divide/2
  Add/1 -> Divide/1
  Sum_F_x [N]/1 -> Product1/1

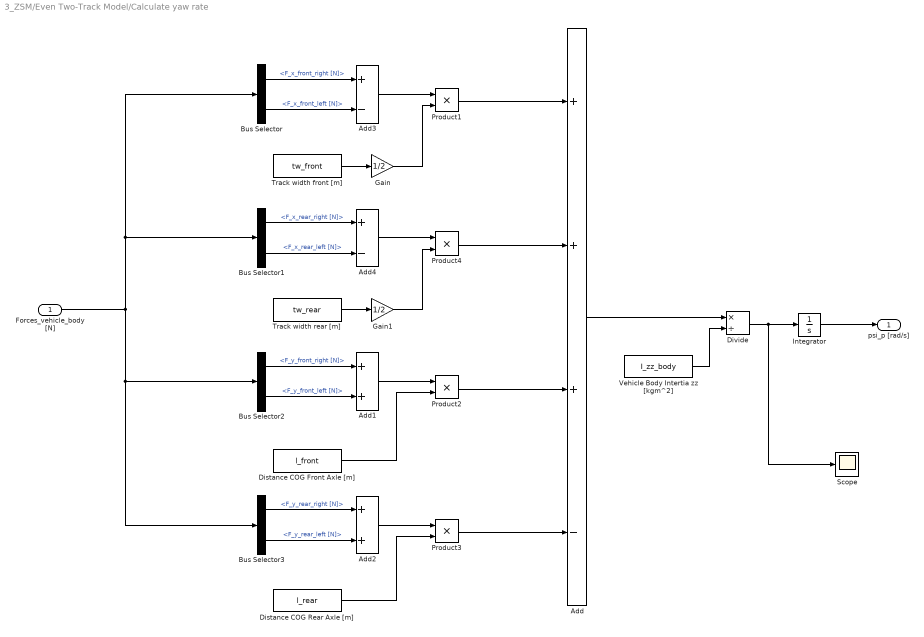
== system 3_ZSM/Even Two-Track Model/Calculate yaw rate ==
  Forces_vehicle_body [N] : Inport
  Add : Sum  Inputs=+++-
  Add1 : Sum
  Add2 : Sum
  Add3 : Sum  Inputs=+-
  Add4 : Sum  Inputs=+-
  Bus Selector : BusSelector  OutputSignals=F_x_front_right [N],F_x_front_left [N]
  Bus Selector1 : BusSelector  OutputSignals=F_x_rear_right [N],F_x_rear_left [N]
  Bus Selector2 : BusSelector  OutputSignals=F_y_front_right [N],F_y_front_left [N]
  Bus Selector3 : BusSelector  OutputSignals=F_y_rear_right [N],F_y_rear_left [N]
  Distance COG Front Axle [m] : Constant  Value=l_front
  Distance COG Rear Axle [m] : Constant  Value=l_rear
  Divide : Product  Inputs=*/
  Gain : Gain  Gain=1/2
  Gain1 : Gain  Gain=1/2
  Integrator : Integrator
  Product{1..4} (4 alike) : Product
  Scope : Scope
  Track width front [m] : Constant  Value=tw_front
  Track width rear [m] : Constant  Value=tw_rear
  Vehicle Body Intertia zz [kgm^2] : Constant  Value=I_zz_body
  psi_p [rad/s] : Outport
  wires:
  Integrator/1 -> psi_p [rad/s]/1
  Bus Selector3/2 -> Add2/2  "<F_y_rear_left [N]>"
  Bus Selector/1 -> Add3/1  "<F_x_front_right [N]>"
  Forces_vehicle_body [N]/1 -> Bus Selector/1, Bus Selector1/1, Bus Selector2/1, Bus Selector3/1
  Vehicle Body Intertia zz [kgm^2]/1 -> Divide/2
  Product3/1 -> Add/4
  Product2/1 -> Add/3
  Product4/1 -> Add/2
  Product1/1 -> Add/1
  Gain1/1 -> Product4/2
  Track width rear [m]/1 -> Gain1/1
  Add4/1 -> Product4/1
  Bus Selector1/2 -> Add4/2  "<F_x_rear_left [N]>"
  Bus Selector1/1 -> Add4/1  "<F_x_rear_right [N]>"
  Gain/1 -> Product1/2
  Track width front [m]/1 -> Gain/1
  Add3/1 -> Product1/1
  Bus Selector/2 -> Add3/2  "<F_x_front_left [N]>"
  Bus Selector3/1 -> Add2/1  "<F_y_rear_right [N]>"
  Add2/1 -> Product3/1
  Add1/1 -> Product2/1
  Bus Selector2/2 -> Add1/2  "<F_y_front_left [N]>"
  Bus Selector2/1 -> Add1/1  "<F_y_front_right [N]>"
  Add/1 -> Divide/1
  Divide/1 -> Scope/1, Integrator/1
  Distance COG Front Axle [m]/1 -> Product2/2
  Distance COG Rear Axle [m]/1 -> Product3/2

== system 3_ZSM/Even Two-Track Model/Determine vehicle body movement in vehicle COS ==
  v [m/s] : Inport
  v_p [m/s^2] : Inport  Port=2
  beta [rad] : Inport  Port=3
  beta_p [rad/s] : Inport  Port=4
  psi_p [rad/s] : Inport  Port=5
  Add : Sum
  Add1 : Sum
  Add2 : Sum  Inputs=+-
  Product{,1..4} (5 alike) : Product
  Trigonometric Function : Trigonometry
  Trigonometric Function1 : Trigonometry  Operator=cos
  a_x [m/s^2] : Outport
  a_y [m/s^2] : Outport  Port=2
  wires:
  beta [rad]/1 -> Trigonometric Function/1, Trigonometric Function1/1
  v_p [m/s^2]/1 -> Product/1, Product2/1
  Trigonometric Function/1 -> Product4/1, Product/2
  beta_p [rad/s]/1 -> Add/1
  psi_p [rad/s]/1 -> Add/2
  Add/1 -> Product1/2
  v [m/s]/1 -> Product1/1
  Product/1 -> Add1/1
  Add1/1 -> a_y [m/s^2]/1
  Add2/1 -> a_x [m/s^2]/1
  Product1/1 -> Product3/2, Product4/2
  Product3/1 -> Add1/2
  Product2/1 -> Add2/1
  Product4/1 -> Add2/2
  Trigonometric Function1/1 -> Product2/2, Product3/1

== system 3_ZSM/Even Two-Track Model/Determine wheel movement ==
  vehicle_velocity [m/s] : Inport
  beta [rad] : Inport  Port=2
  psi_p [rad/s] : Inport  Port=3
  Vehicle Bus In : Inport  Port=4
  Calculate slip angle front left : Subsystem
  Calculate slip angle front right : Subsystem
  Calculate slip angle rear left : Subsystem
  Calculate slip angle rear right : Subsystem
  Precalculation : Subsystem
  alpha_front_right [rad] : Outport
  alpha_front_left [rad] : Outport  Port=2
  alpha_rear_right [rad] : Outport  Port=3
  alpha_rear_left [rad] : Outport  Port=4
  wires:
  Calculate slip angle rear right/1(alpha_rear_right [rad]) -> alpha_rear_right [rad]/1
  Precalculation/1(Input Signals) -> Calculate slip angle front left/2(Calculated Inputs), Calculate slip angle rear right/2(Calculated Inputs), Calculate slip angle rear left/2(Calculated Inputs), Calculate slip angle front right/2(Calculated Inputs)
  Vehicle Bus In/1 -> Calculate slip angle front left/1(Vehicle Bus), Calculate slip angle front right/1(Vehicle Bus), Calculate slip angle rear left/1(Vehicle Bus), Calculate slip angle rear right/1(Vehicle Bus)
  Calculate slip angle rear left/1(alpha_rear_left [rad]) -> alpha_rear_left [rad]/1
  Calculate slip angle front right/1(alpha_front_right [rad]) -> alpha_front_right [rad]/1
  Calculate slip angle front left/1(alpha_front_left [rad]) -> alpha_front_left [rad]/1
  psi_p [rad/s]/1 -> Precalculation/3(psi_p [rad/s])
  beta [rad]/1 -> Precalculation/2(beta [rad])
  vehicle_velocity [m/s]/1 -> Precalculation/1(vehicle_velocity [m/s])

== system 3_ZSM/Tire/Tire front left ==
  F_powertrain [N] : Inport
  Wheel_Bus : Inport  Port=2
  nu_v_l [-] : Inport  Port=3
  Bus Creator : BusCreator  Inputs=4
  Bus Selector1 : BusSelector  OutputSignals=alpha_v_l [rad],F_z_v_l [N]
  Fcn : Fcn  Expr=u(1)<=u(2)
  Kammscher Kreis : Subsystem
  Mux : Mux  Inputs=2
  Pacejka Front Left : Subsystem
  Switch : Switch  Criteria=u2 > Threshold
  Tire_front_left : Outport
  wires:
  Bus Creator/1 -> Tire_front_left/1
  Wheel_Bus/1 -> Bus Selector1/1
  Bus Selector1/1 -> Pacejka Front Left/2(alpha_v_in [rad])  "<alpha_v_l [rad]>"
  nu_v_l [-]/1 -> Pacejka Front Left/1(nu_v_l [-])
  Bus Selector1/2 -> Pacejka Front Left/3(F_z_v_l [N]), Kammscher Kreis/1(F_z_FL [N])  "<F_z_v_l [N]>"
  F_powertrain [N]/1 -> Kammscher Kreis/2(F_x_FL [N]), Bus Creator/1  "F_x_v_l [N]"
  Pacejka Front Left/1(F_y_v_l [N]) -> Mux/1, Switch/1  "F_y_v_l [N]"
  Fcn/1 -> Switch/2
  Mux/1 -> Fcn/1
  Kammscher Kreis/1(F_y_v_l_max [N]) -> Mux/2, Switch/3, Bus Creator/3  "F_y_v_l_max [N]"
  Switch/1 -> Bus Creator/2  "F_y_v_l [N]"
  Kammscher Kreis/2(F_v_l_max [N]) -> Bus Creator/4  "F_v_l_max [N]"

== system 3_ZSM/Tire/Tire front right ==
  F_powertrain [N] : Inport
  Wheel_Bus : Inport  Port=2
  nu_v_r [-] : Inport  Port=3
  Bus Creator : BusCreator  Inputs=4
  Bus Selector1 : BusSelector  OutputSignals=alpha_v_r [rad],F_z_v_r [N]
  Fcn : Fcn  Expr=u(1)<=u(2)
  Kammscher Kreis : Subsystem
  Mux : Mux  Inputs=2
  Pacejka Front right : Subsystem
  Switch : Switch  Criteria=u2 > Threshold
  Tire_front_right : Outport
  wires:
  Bus Creator/1 -> Tire_front_right/1
  Wheel_Bus/1 -> Bus Selector1/1
  Bus Selector1/1 -> Pacejka Front right/2(alpha_v_in [rad])  "<alpha_v_r [rad]>"
  nu_v_r [-]/1 -> Pacejka Front right/1(nu_v_r [-])
  Bus Selector1/2 -> Kammscher Kreis/1(F_z_v_r [N]), Pacejka Front right/3(F_z_v_r [N])  "<F_z_v_r [N]>"
  F_powertrain [N]/1 -> Kammscher Kreis/2(F_x_v_r [N]), Bus Creator/1  "F_x_v_r [N]"
  Pacejka Front right/1(F_y_v_r [N]) -> Mux/1, Switch/1
  Fcn/1 -> Switch/2
  Mux/1 -> Fcn/1
  Kammscher Kreis/1(F_y_v_r_max [N]) -> Mux/2, Switch/3, Bus Creator/3  "F_y_v_r_max [N]"
  Switch/1 -> Bus Creator/2  "F_y_v_r [N]"
  Kammscher Kreis/2(F_v_r_max [N]) -> Bus Creator/4  "F_v_r_max [N]"

== system 3_ZSM/Tire/Tire rear left ==
  F_powertrain [N] : Inport
  Wheel_Bus : Inport  Port=2
  nu_h_l [-] : Inport  Port=3
  Bus Creator : BusCreator  Inputs=4
  Bus Selector1 : BusSelector  OutputSignals=alpha_h_l [rad],F_z_h_l [N]
  Fcn : Fcn  Expr=u(1)<=u(2)
  Kammscher Kreis : Subsystem
  Mux : Mux  Inputs=2
  Pacejka Front Left : Subsystem
  Switch : Switch  Criteria=u2 > Threshold
  Tire_rear_left : Outport
  wires:
  Bus Creator/1 -> Tire_rear_left/1
  Wheel_Bus/1 -> Bus Selector1/1
  Bus Selector1/1 -> Pacejka Front Left/2(alpha_h_in [rad])  "<alpha_h_l [rad]>"
  nu_h_l [-]/1 -> Pacejka Front Left/1(nu_h_l [-])
  Bus Selector1/2 -> Kammscher Kreis/1(F_z_h_l [N]), Pacejka Front Left/3(F_z_h_l [N])  "<F_z_h_l [N]>"
  F_powertrain [N]/1 -> Kammscher Kreis/2(F_x_h_l [N]), Bus Creator/1  "F_x_h_l [N]"
  Pacejka Front Left/1(F_y_h_l [N]) -> Mux/1, Switch/1
  Fcn/1 -> Switch/2
  Mux/1 -> Fcn/1
  Kammscher Kreis/1(F_y_h_l_max [N]) -> Mux/2, Switch/3, Bus Creator/3  "F_y_h_l_max [N]"
  Switch/1 -> Bus Creator/2  "F_y_h_l [N]"
  Kammscher Kreis/2(F_h_l_max [N]) -> Bus Creator/4  "F_h_l_max [N]"

== system 3_ZSM/Tire/Tire rear right ==
  F_powertrain [N] : Inport
  Wheel_Bus : Inport  Port=2
  nu_h_r [-] : Inport  Port=3
  Bus Creator : BusCreator  Inputs=4
  Bus Selector1 : BusSelector  OutputSignals=alpha_h_l [rad],F_z_h_r [N]
  Fcn : Fcn  Expr=u(1)<=u(2)
  Kammscher Kreis : Subsystem
  Mux : Mux  Inputs=2
  Pacejka Front Left : Subsystem
  Switch : Switch  Criteria=u2 > Threshold
  Tire_front_left : Outport
  wires:
  Bus Creator/1 -> Tire_front_left/1
  Wheel_Bus/1 -> Bus Selector1/1
  Bus Selector1/1 -> Pacejka Front Left/2(alpha_h_in [rad])  "<alpha_h_l [rad]>"
  nu_h_r [-]/1 -> Pacejka Front Left/1(nu_h_r [-])
  Bus Selector1/2 -> Kammscher Kreis/1(F_z_h_r [N]), Pacejka Front Left/3(F_z_h_r [N])  "<F_z_h_r [N]>"
  F_powertrain [N]/1 -> Kammscher Kreis/2(F_x_h_r [N]), Bus Creator/1  "F_x_h_r [N]"
  Pacejka Front Left/1(F_y_h_r [N]) -> Mux/1, Switch/1
  Fcn/1 -> Switch/2
  Mux/1 -> Fcn/1
  Kammscher Kreis/1(F_y_h_r_max [N]) -> Mux/2, Switch/3, Bus Creator/3  "F_y_h_r_max [N]"
  Switch/1 -> Bus Creator/2  "F_y_h_r [N]"
  Kammscher Kreis/2(F_h_r_max [N]) -> Bus Creator/4  "F_h_r_max [N]"

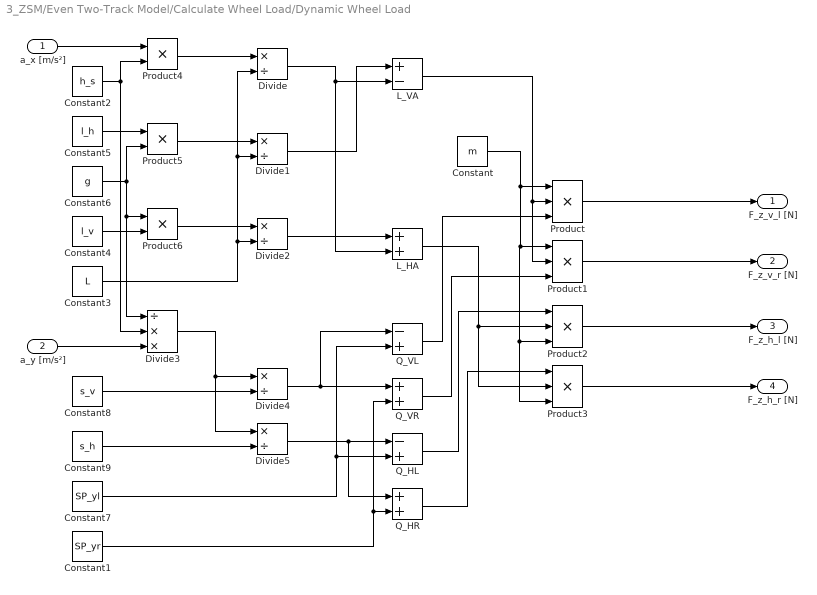
== system 3_ZSM/Even Two-Track Model/Calculate Wheel Load/Dynamic Wheel Load ==
  a_x [m/s²] : Inport
  a_y [m/s²] : Inport  Port=2
  Constant : Constant  Value=m
  Constant1 : Constant  Value=SP_yr
  Constant2 : Constant  Value=h_s
  Constant3 : Constant  Value=L
  Constant4 : Constant  Value=l_v
  Constant5 : Constant  Value=l_h
  Constant6 : Constant  Value=g
  Constant7 : Constant  Value=SP_yl
  Constant8 : Constant  Value=s_v
  Constant9 : Constant  Value=s_h
  Divide{,1..2,4..5} (5 alike) : Product  Inputs=*/
  Divide3 : Product  Inputs=/**
  L_HA : Sum
  L_VA : Sum  Inputs=+-
  Product{,1..3} (4 alike) : Product  Inputs=3
  Product4 : Product
  Product5 : Product
  Product6 : Product
  Q_HL : Sum  Inputs=-+
  Q_HR : Sum
  Q_VL : Sum  Inputs=-+
  Q_VR : Sum
  F_z_v_l [N] : Outport
  F_z_v_r [N] : Outport  Port=2
  F_z_h_l [N] : Outport  Port=3
  F_z_h_r [N] : Outport  Port=4
  wires:
  Q_VL/1 -> Product/3
  Q_HL/1 -> Product2/1
  Divide5/1 -> Q_HR/1, Q_HL/1
  L_VA/1 -> Product1/2, Product/2
  L_HA/1 -> Product2/2, Product3/2
  Q_HR/1 -> Product3/1
  Q_VR/1 -> Product1/3
  a_y [m/s²]/1 -> Divide3/3
  Constant8/1 -> Divide4/2
  Constant9/1 -> Divide5/2
  Divide3/1 -> Divide5/1, Divide4/1
  Divide4/1 -> Q_VR/1, Q_VL/1
  Product/1 -> F_z_v_l [N]/1
  Constant2/1 -> Divide3/2, Product4/2
  Constant/1 -> Product1/1, Product2/3, Product3/3, Product/1
  Constant3/1 -> Divide/2, Divide1/2, Divide2/2
  Constant5/1 -> Product5/1
  Product6/1 -> Divide2/1
  Product1/1 -> F_z_v_r [N]/1
  Product4/1 -> Divide/1
  Constant6/1 -> Divide3/1, Product6/1, Product5/2
  Product5/1 -> Divide1/1
  Constant4/1 -> Product6/2
  Divide/1 -> L_HA/2, L_VA/2
  Divide1/1 -> L_VA/1
  Product2/1 -> F_z_h_l [N]/1
  Product3/1 -> F_z_h_r [N]/1
  Divide2/1 -> L_HA/1
  a_x [m/s²]/1 -> Product4/1
  Constant1/1 -> Q_VR/2, Q_HR/2
  Constant7/1 -> Q_HL/2, Q_VL/2

== system 3_ZSM/Even Two-Track Model/Calculate Wheel Load/Static Wheel Load ==
  Constant10 : Constant  Value=g
  Constant11 : Constant  Value=m_vl
  Constant12 : Constant  Value=m_vr
  Constant13 : Constant  Value=m_hl
  Constant14 : Constant  Value=m_hr
  Product{7..10} (4 alike) : Product
  F_z_v_l [N] : Outport
  F_z_v_r [N] : Outport  Port=2
  F_z_h_l [N] : Outport  Port=3
  F_z_h_r [N] : Outport  Port=4
  wires:
  Constant10/1 -> Product10/1, Product9/1, Product8/1, Product7/1
  Constant11/1 -> Product7/2
  Constant14/1 -> Product10/2
  Constant13/1 -> Product9/2
  Constant12/1 -> Product8/2
  Product8/1 -> F_z_v_r [N]/1
  Product7/1 -> F_z_v_l [N]/1
  Product9/1 -> F_z_h_l [N]/1
  Product10/1 -> F_z_h_r [N]/1

== system 3_ZSM/Even Two-Track Model/Calculate forces on vehicle body/Transform Wheel-COS to Vehicle-COS (front left) ==
  F_x_wheel_COS [N] : Inport
  F_y_wheel_COS [N] : Inport  Port=2
  Wheel_steering_angle [rad] : Inport  Port=3
  Add : Sum
  Product{,1..3} (4 alike) : Product
  Subtract : Sum  Inputs=+-
  Trigonometric Function : Trigonometry
  Trigonometric Function1 : Trigonometry  Operator=cos
  F_x_vehicle_COS [N] : Outport
  F_y_vehicle_COS [N] : Outport  Port=2
  wires:
  Wheel_steering_angle [rad]/1 -> Trigonometric Function1/1, Trigonometric Function/1
  Product2/1 -> Add/1
  Product/1 -> Subtract/1
  Product1/1 -> Subtract/2
  Product3/1 -> Add/2
  F_x_wheel_COS [N]/1 -> Product2/1, Product/1
  Trigonometric Function1/1 -> Product/2, Product3/2
  F_y_wheel_COS [N]/1 -> Product3/1, Product1/1
  Trigonometric Function/1 -> Product2/2, Product1/2
  Add/1 -> F_y_vehicle_COS [N]/1
  Subtract/1 -> F_x_vehicle_COS [N]/1

== system 3_ZSM/Even Two-Track Model/Calculate forces on vehicle body/Transform Wheel-COS to Vehicle-COS (front right) ==
  F_x_wheel_COS [N] : Inport
  F_y_wheel_COS [N] : Inport  Port=2
  Wheel_steering_angle [rad] : Inport  Port=3
  Add : Sum
  Product{,1..3} (4 alike) : Product
  Subtract : Sum  Inputs=+-
  Trigonometric Function : Trigonometry
  Trigonometric Function1 : Trigonometry  Operator=cos
  F_x_vehicle_COS [N] : Outport
  F_y_vehicle_COS [N] : Outport  Port=2
  wires:
  Add/1 -> F_y_vehicle_COS [N]/1
  Subtract/1 -> F_x_vehicle_COS [N]/1
  Wheel_steering_angle [rad]/1 -> Trigonometric Function1/1, Trigonometric Function/1
  Product2/1 -> Add/1
  Product/1 -> Subtract/1
  Product1/1 -> Subtract/2
  Product3/1 -> Add/2
  F_x_wheel_COS [N]/1 -> Product2/1, Product/1
  Trigonometric Function1/1 -> Product/2, Product3/2
  F_y_wheel_COS [N]/1 -> Product3/1, Product1/1
  Trigonometric Function/1 -> Product2/2, Product1/2

== system 3_ZSM/Even Two-Track Model/Calculate forces on vehicle body/Transform Wheel-COS to Vehicle-COS (rear left) ==
  F_x_wheel_COS [N] : Inport
  F_y_wheel_COS [N] : Inport  Port=2
  Wheel_steering_angle [rad] : Inport  Port=3
  Add : Sum
  Product{,1..3} (4 alike) : Product
  Subtract : Sum  Inputs=+-
  Trigonometric Function : Trigonometry
  Trigonometric Function1 : Trigonometry  Operator=cos
  F_x_vehicle_COS [N] : Outport
  F_y_vehicle_COS [N] : Outport  Port=2
  wires:
  Wheel_steering_angle [rad]/1 -> Trigonometric Function1/1, Trigonometric Function/1
  Product2/1 -> Add/1
  Product/1 -> Subtract/1
  Product1/1 -> Subtract/2
  Product3/1 -> Add/2
  F_x_wheel_COS [N]/1 -> Product2/1, Product/1
  Trigonometric Function1/1 -> Product/2, Product3/2
  F_y_wheel_COS [N]/1 -> Product3/1, Product1/1
  Trigonometric Function/1 -> Product2/2, Product1/2
  Subtract/1 -> F_x_vehicle_COS [N]/1
  Add/1 -> F_y_vehicle_COS [N]/1

== system 3_ZSM/Even Two-Track Model/Calculate forces on vehicle body/Transform Wheel-COS to Vehicle-COS (rear right) ==
  F_x_wheel_COS [N] : Inport
  F_y_wheel_COS [N] : Inport  Port=2
  Wheel_steering_angle [rad] : Inport  Port=3
  Add : Sum
  Product{,1..3} (4 alike) : Product
  Subtract : Sum  Inputs=+-
  Trigonometric Function : Trigonometry
  Trigonometric Function1 : Trigonometry  Operator=cos
  F_x_vehicle_COS [N] : Outport
  F_y_vehicle_COS [N] : Outport  Port=2
  wires:
  Wheel_steering_angle [rad]/1 -> Trigonometric Function1/1, Trigonometric Function/1
  Product2/1 -> Add/1
  Product/1 -> Subtract/1
  Product1/1 -> Subtract/2
  Product3/1 -> Add/2
  F_x_wheel_COS [N]/1 -> Product2/1, Product/1
  Trigonometric Function1/1 -> Product/2, Product3/2
  F_y_wheel_COS [N]/1 -> Product3/1, Product1/1
  Trigonometric Function/1 -> Product2/2, Product1/2
  Add/1 -> F_y_vehicle_COS [N]/1
  Subtract/1 -> F_x_vehicle_COS [N]/1

== system 3_ZSM/Even Two-Track Model/Determine wheel movement/Calculate slip angle front left ==
  Vehicle Bus : Inport
  Calculated Inputs : Inport  Port=2
  Bus Selector : BusSelector  OutputSignals=Steering_Bus.Delta_v_l
  Bus Selector1 : BusSelector  OutputSignals=v_beta_sin,psi_p_l_front
  Bus Selector2 : BusSelector  OutputSignals=v_beta_cos,psi_p_tw_front
  Divide : Product  Inputs=*/
  Sum : Sum  Inputs=+-  SaturateOnIntegerOverflow=on
  Sum1 : Sum  Inputs=+-  SaturateOnIntegerOverflow=on
  Sum2 : Sum  SaturateOnIntegerOverflow=on
  Trigonometric Function : Trigonometry  Operator=atan
  alpha_front_left [rad] : Outport
  wires:
  Bus Selector2/1 -> Sum1/1  "<v_beta_cos>"
  Calculated Inputs/1 -> Bus Selector1/1, Bus Selector2/1
  Bus Selector2/2 -> Sum1/2  "<psi_p_tw_front>"
  Sum1/1 -> Divide/2
  Bus Selector1/2 -> Sum2/2  "<psi_p_l_front>"
  Bus Selector1/1 -> Sum2/1  "<v_beta_sin>"
  Sum2/1 -> Divide/1
  Trigonometric Function/1 -> Sum/2
  Divide/1 -> Trigonometric Function/1
  Vehicle Bus/1 -> Bus Selector/1
  Sum/1 -> alpha_front_left [rad]/1
  Bus Selector/1 -> Sum/1  "<Delta_v_l>"

== system 3_ZSM/Even Two-Track Model/Determine wheel movement/Calculate slip angle front right ==
  Vehicle Bus : Inport
  Calculated Inputs : Inport  Port=2
  Bus Selector : BusSelector  OutputSignals=Steering_Bus.Delta_v_r
  Bus Selector1 : BusSelector  OutputSignals=v_beta_sin,psi_p_l_front
  Bus Selector2 : BusSelector  OutputSignals=v_beta_cos,psi_p_tw_front
  Divide : Product  Inputs=*/
  Sum : Sum  Inputs=+-  SaturateOnIntegerOverflow=on
  Sum1 : Sum  SaturateOnIntegerOverflow=on
  Sum2 : Sum  SaturateOnIntegerOverflow=on
  Trigonometric Function : Trigonometry  Operator=atan
  alpha_front_right [rad] : Outport
  wires:
  Bus Selector2/1 -> Sum1/1  "<v_beta_cos>"
  Calculated Inputs/1 -> Bus Selector1/1, Bus Selector2/1
  Bus Selector2/2 -> Sum1/2  "<psi_p_tw_front>"
  Sum1/1 -> Divide/2
  Bus Selector1/2 -> Sum2/2  "<psi_p_l_front>"
  Bus Selector1/1 -> Sum2/1  "<v_beta_sin>"
  Sum2/1 -> Divide/1
  Trigonometric Function/1 -> Sum/2
  Divide/1 -> Trigonometric Function/1
  Vehicle Bus/1 -> Bus Selector/1
  Sum/1 -> alpha_front_right [rad]/1
  Bus Selector/1 -> Sum/1  "<Delta_v_r>"
